simulink model "chap6_5sim"  (Simulink 5.0)
settings: Solver=ode45  StartTime=0.0  StopTime=50
settings Model: LastModifiedBy=Administrator  ExtModeTrigMode=oneshot  ExtModeArmWhenConnect=off  LimitDataPoints=off  BooleanDataType=off

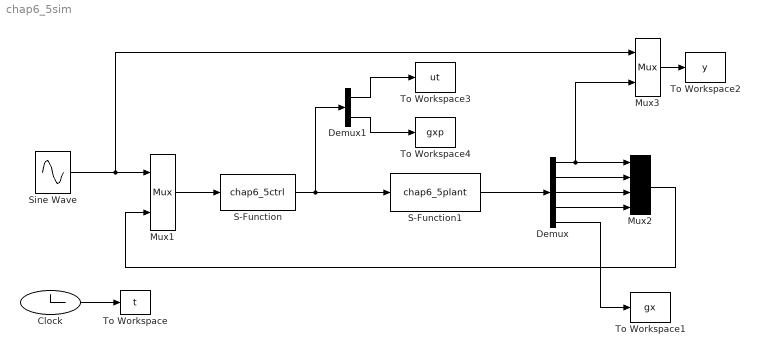
== system chap6_5sim ==
  Clock : Clock
  Demux : Demux  Outputs=5
  Demux1 : Demux  Outputs=2
  Mux1 : Mux  Inputs=2
  Mux2 : Mux
  Mux3 : Mux  Inputs=2
  S-Function : S-Function  FunctionName=chap6_5ctrl
  S-Function1 : S-Function  FunctionName=chap6_5plant
  Sine Wave : Sin  SampleTime=0
  To Workspace : ToWorkspace  VariableName=t  SampleTime=-1  SaveFormat=Array
  To Workspace1 : ToWorkspace  VariableName=gx  SampleTime=-1  SaveFormat=Array
  To Workspace2 : ToWorkspace  VariableName=y  SampleTime=-1  SaveFormat=Array
  To Workspace3 : ToWorkspace  VariableName=ut  SampleTime=-1  SaveFormat=Array
  To Workspace4 : ToWorkspace  VariableName=gxp  SampleTime=-1  SaveFormat=Array
  wires:
  Clock/1 -> To Workspace/1
  S-Function/1 -> S-Function1/1, Demux1/1
  Sine Wave/1 -> Mux1/1, Mux3/1
  S-Function1/1 -> Demux/1
  Mux1/1 -> S-Function/1
  Demux/1 -> Mux3/2, Mux2/1
  Mux3/1 -> To Workspace2/1
  Demux/2 -> Mux2/2
  Demux/3 -> Mux2/3
  Mux2/1 -> Mux1/2
  Demux/5 -> To Workspace1/1
  Demux/4 -> Mux2/4
  Demux1/1 -> To Workspace3/1
  Demux1/2 -> To Workspace4/1
